simulink model "ESC_Example"  (Simulink 8.3)
settings: Solver=ode45  StartTime=0.0  StopTime=5  MaxStep=0.001  RelTol=1e-3
model workspace (MAT data in the model file):
  Cf = 38925
  Cr = 38255
  Izz = 5428
  K = 19
  X = [0 0.000200950914521 0.00120570548712 0.00622947835014 0.0313483426652 0.0646816759986 0.0980150093319 0.131348342665 0.164681675999 0.198015009332 0.231348342665 0.264681675999 ... (5155 elements, 5155x1)]
  Y = [0 0 0 0 0 0 0 0 0 0 0 0 ... (5155 elements, 5155x1)]
  deltaf = [0 0 0 0 0 0 0 0 0 0 0 0 ... (5155 elements, 5155x1)]
  frame = 100
  imanual = 0
  lf = 1.488
  lr = 1.712
  m = 2045
  mu = 0.9
  ncar = 10
  psi = [0 0 0 0 0 0 0 0 0 0 0 0 ... (5155 elements, 5155x1)]
  scale = 2
  tout = [0 6.02852743562e-06 3.61711646137e-05 0.000186884350504 0.000940450279957 0.00194045027996 0.00294045027996 0.00394045027996 0.00494045027996 0.00594045027996 0.00694045027996 0.00794045027996 ... (5155 elements, 5155x1)]
  yout = [0 0.000200950914521 0.00120570548712 0.00622947835014 0.0313483426652 0.0646816759986 0.0980150093319 0.131348342665 0.164681675999 0.198015009332 0.231348342665 0.264681675999 ... (20620 elements, 5155x4)]
PreLoadFcn:
  | load('ESC_Example.mat');
StopFcn:
  | X = yout(:,1);
  | Y = yout(:,2);
  | psi = yout(:,3);
  | deltaf = yout(:,4);
  | frame = 100;
  | imanual = 0;
  | scale = 2;
  | ncar = 10;
  | 
  | anim_tracking_ESC(X,Y,psi,tout,scale,deltaf,frame,imanual)
undefined symbols (not defined in the file): sigbuilder_block
libraries: simulink x1
settings Model: Creator=Park  LastModifiedBy=user
settings DataIOCC: LimitDataPoints=off
settings OptimizationCC: ExpressionDepthLimit=2147483647
settings DebuggingCC: FcnCallInpInsideContextMsg=UseLocalSettings  FrameProcessingCompatibilityMsg=error
settings ConfigComp: CovMetricSettings=dw  CovHtmlReporting=on  CovSaveCumulativeToWorkspaceVar=on  CovSaveSingleToWorkspaceVar=on  CovModelRefEnable=Off  CovExternalEMLEnable=off

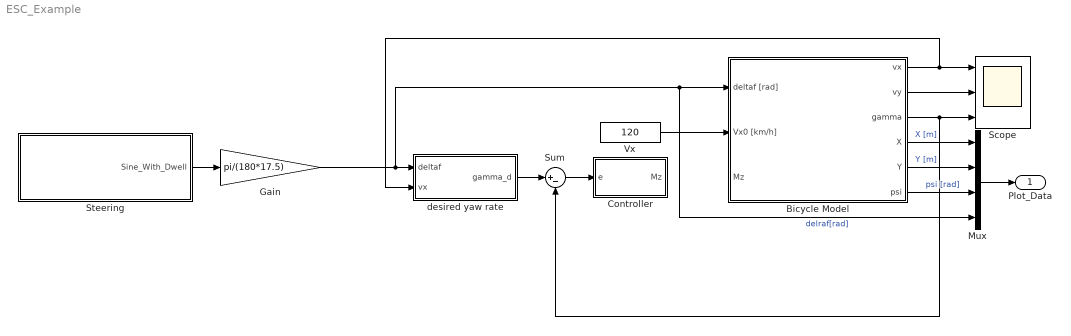
== system ESC_Example ==
  Bicycle Model : Subsystem
  Controller : Subsystem  TreatAsAtomicUnit=on
  Gain : Gain  Gain=pi/(180*17.5)
  Mux : Mux
  Scope : Scope  NumInputPorts=3
  Steering : Subsystem  Tag=STV Subsys  LoadFcn=sigbuilder_block('load');  StartFcn=sigbuilder_block('start');  StopFcn=sigbuilder_block('stop');  ClipboardFcn=sigbuilder_block('clipboard');  mask(Sigbuilder block){}
      mask help: Simulink:masks:SigbuilderBlock_MD
      mask init:
      | if ~strcmp(get_param(bdroot(gcbh),'SimulationStatus'),'stopped') tuvar = sigbuilder_block('maskInit'); end
      settings: CopyFcn=sigbuilder_block('copy');  DeleteFcn=sigbuilder_block('delete');  ModelCloseFcn=sigbuilder_block('modelClose');  PreSaveFcn=sigbuilder_block('preSave');  PauseFcn=sigbuilder_block('pause');  ContinueFcn=sigbuilder_block('continue');  NameChangeFcn=sigbuilder_block('namechange');  OpenFcn=sigbuilder_block('open',[0 29.7931 635.586 392.276 ]);  CloseFcn=sigbuilder_block('close');
      mask Display: plot(0, 0, 100, 100,[2, 2, 32, 32, 2], [68, 8, 8, 68, 68],[32, 2], [38, 38], [32, 19, 2],[53, 60, 44], [32, 17, 17, 2],[16, 16, 31, 31]);txt = getActiveGroup(gcbh);text(2, 100, txt,'verticalAlignment', 'top');
  Sum : Sum  Inputs=|+-
  Vx : Constant  Value=120
  desired yaw rate : Subsystem
  Plot_Data : Outport
  wires:
  Steering/1(Sine_With_Dwell) -> Gain/1
  Bicycle Model/4(X) -> Mux/1  "X [m]"
  Bicycle Model/5(Y) -> Mux/2  "Y [m]"
  Bicycle Model/6(psi) -> Mux/3  "psi [rad]"
  Mux/1 -> Plot_Data/1
  Bicycle Model/1(vx) -> desired yaw rate/2(vx), Scope/1
  Bicycle Model/2(vy) -> Scope/2
  Bicycle Model/3(gamma) -> Sum/2, Scope/3
  Gain/1 -> Mux/4, Bicycle Model/1(deltaf [rad]), desired yaw rate/1(deltaf)  "delraf[rad]"
  desired yaw rate/1(gamma_d) -> Sum/1
  Sum/1 -> Controller/1(e)
  Vx/1 -> Bicycle Model/2(Vx0 [km/h])

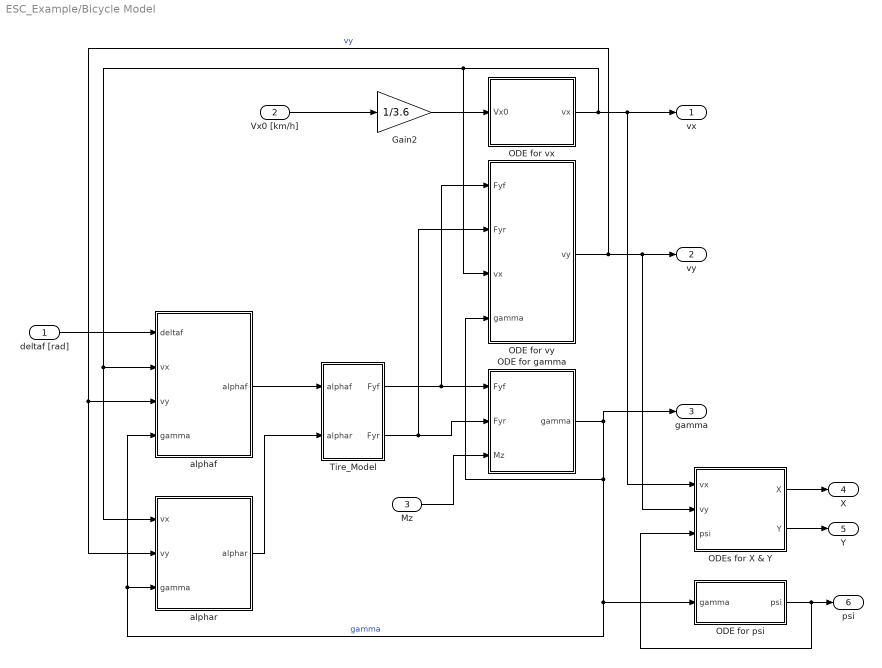
== system ESC_Example/Bicycle Model ==
  deltaf [rad] : Inport
  Vx0 [km/h] : Inport  Port=2
  Mz : Inport  Port=3
  Gain2 : Gain  Gain=1/3.6
  ODE for gamma : Subsystem
  ODE for psi : Subsystem
  ODE for vx : Subsystem
  ODE for vy : Subsystem
  ODEs for X & Y : Subsystem
  Tire_Model : Subsystem  Variant=on
  alphaf : Subsystem
  alphar : Subsystem
  vx : Outport
  vy : Outport  Port=2
  gamma : Outport  Port=3
  X : Outport  Port=4
  Y : Outport  Port=5
  psi : Outport  Port=6
  wires:
  alphaf/1(alphaf) -> Tire_Model/1(alphaf)
  alphar/1(alphar) -> Tire_Model/2(alphar)
  Tire_Model/1(Fyf) -> ODE for gamma/1(Fyf), ODE for vy/1(Fyf)
  Tire_Model/2(Fyr) -> ODE for gamma/2(Fyr), ODE for vy/2(Fyr)
  ODE for gamma/1(gamma) -> gamma/1, ODE for vy/4(gamma), alphar/3(gamma), alphaf/4(gamma), ODE for psi/1(gamma)  "gamma"
  ODE for vy/1(vy) -> ODEs for X & Y/2(vy), vy/1, alphaf/3(vy), alphar/2(vy)  "vy"
  ODE for vx/1(vx) -> alphaf/2(vx), alphar/1(vx), ODE for vy/3(vx), ODEs for X & Y/1(vx), vx/1
  ODE for psi/1(psi) -> ODEs for X & Y/3(psi), psi/1
  deltaf [rad]/1 -> alphaf/1(deltaf)
  ODEs for X & Y/1(X) -> X/1
  ODEs for X & Y/2(Y) -> Y/1
  Vx0 [km/h]/1 -> Gain2/1
  Gain2/1 -> ODE for vx/1(Vx0)
  Mz/1 -> ODE for gamma/3(Mz)

== system ESC_Example/Controller ==
  e : Inport
  PID Controller : simulink/Continuous/PID Controller  Controller=PID  TimeDomain=Continuous-time  SampleTime=-1  IntegratorMethod=Forward Euler  FilterMethod=Forward Euler  Form=Parallel  P=108153.175289364  I=433866.001986902  D=-1959.17350386418  N=55.2034697672503  InitialConditionSource=internal  InitialConditionForIntegrator=0  InitialConditionForFilter=0  ExternalReset=none  LimitOutput=off  UpperSaturationLimit=inf  LowerSaturationLimit=-inf  LinearizeAsGain=on  AntiWindupMode=none  Kb=1  TrackingMode=off  Kt=1  PParamMin=[]  PParamMax=[]  IParamMin=[]  IParamMax=[]  DParamMin=[]  DParamMax=[]  NParamMin=[]  NParamMax=[]  KbParamMin=[]  KbParamMax=[]  KtParamMin=[]  KtParamMax=[]  POutMin=[]  POutMax=[]  IOutMin=[]  IOutMax=[]  DOutMin=[]  DOutMax=[]  NOutMin=[]  NOutMax=[]  KbOutMin=[]  KbOutMax=[]  KtOutMin=[]  KtOutMax=[]  IntegratorOutMin=[]  IntegratorOutMax=[]  FilterOutMin=[]  FilterOutMax=[]  SumOutMin=[]  SumOutMax=[]  SumI1OutMin=[]  SumI1OutMax=[]  SumI2OutMin=[]  SumI2OutMax=[]  SumI3OutMin=[]  SumI3OutMax=[]  SumDOutMin=[]  SumDOutMax=[]  SaturationOutMin=[]  SaturationOutMax=[]  IntegratorContinuousStateAttributes=''  IntegratorStateMustResolveToSignalObject=off  IntegratorRTWStateStorageClass=Auto  FilterContinuousStateAttributes=''  FilterStateMustResolveToSignalObject=off  FilterRTWStateStorageClass=Auto
  Mz : Outport
  wires:
  e/1 -> PID Controller/1
  PID Controller/1 -> Mz/1

== system ESC_Example/Steering ==
  Demux : Demux  Tag=STV Demux  Outputs=1
  FromWs : FromWorkspace  Tag=STV FromWs  VariableName=tuvar  SampleTime=0  SigBuilderData=DataTag1  VnvData=DataTag2
      SigBuilderData=|
      | common.afterFinalStr = 'Extrapolate'
      | common.sampleTime = 0
      | dataSet.timeRange = [0 10]
      | dataSet.name = 'Sine_With_Dwell'
      | sbobj.Groups.Name = 'Sine_With_Dwell'
      | sbobj.Groups.Signals.Name = 'Sine_With_Dwell'
      | sbobj.Groups.Signals.XData = [0 1 1.01 1.02 1.03 1.04 1.05 1.06 1.07 1.08 1.09 1.1 1.11 1.12 1.13 1.14 1.15 1.16 1.17 1.18 1.19 1.2 1.21 1.22 1.23 1.24 1.25 1.26 1.27 1.28 1.29 1.3 1.31 1.32 1.33 1.34 1.35 1.36 1.37 1.38 1.39 1.4 1.41 1.42 1.43 1.44 1.45 1.46 1.47 1.48 1.49 1.5 1.51 1.52 1.53 1.54 1.55 1.56 1.57 1.58 1.59 1.6 1.61 1.62 1.63 1.64 1.65 1.66 1.67 1.68 1.69 1.7 1.71 1.72 1.73 1.74 1.75 1.76 1.77 1.78 1.79 1.8 1.81 1.82 1.83 1.84 1.85 1.86 1.87 1.88 1.89 1.9 1.91 1.92 1.93 1.94 1.95 1.96 1.97 1.98 1.99 2 2.01 2.02 2.03 2.04 2.05 2.06 2.07 2.071 2.57 2.58 2.59 2.6 2.61 2.62 2.63 2.64 2.65 2.66 2.67 2.68 2.69 2.7 2.71 2.72 2.73 2.74 2.75 2.76 2.77 2.78 2.79 2.8 2.81 2.82 2.83 2.84 2.85 2.86 2.87 2.88 2.89 2.9 2.91 2.92 2.927 10]
      | sbobj.Groups.Signals.YData = [0 0 11.87139195 23.71982307 35.52237696 47.25622593 58.89867518 70.4272067 81.8195228 93.05358926 104.1076779 114.9604087 125.5907911 135.9782644 146.1027381 155.9446299 165.4849046 174.7051097 183.5874123 192.1146329 200.2702787 208.0385756 215.4044987 222.3538014 228.8730428 234.9496137 240.5717616 245.7286121 250.4101914 254.6074448 258.312254 261.5174535 264.2168442 266.405205 268.0783032 269.232903 269.8667714 269.978682 269.5684185 268.6367747 267.185552 265.2175577 262.736598 259.7474714 256.2559592 252.2688144 247.7937489 242.839418 237.4154037 231.5321972 225.2011772 218.4345885 211.2455189 203.6478728 195.6563451 187.2863925 178.5542037 169.4766675 160.0713414 150.3564165 140.3506825 130.073492 119.5447224 108.7847376 97.81434902 86.65477466 75.32759864 63.85472919 52.25835638 40.56090906 28.78501166 16.95344028 5.089078724 -6.78512577 -18.64620695 -30.47122392 -42.23730557 -53.92169474 -65.50179231 -76.95520086 -88.25976801 -99.39362922 -110.3352502 -121.0634684 -131.5575339 -141.7971501 -151.762512 -161.4343455 -170.7939437 -179.8232042 -188.5046631 -196.8215294 -204.7577172 -212.2978767 -219.4274244 -226.1325708 -232.4003474 -238.2186312 -243.5761691 -248.4625988 -252.8684694 -256.7852594 -260.2053932 -263.1222557 -265.5302054 -267.4245849 -268.8017304 -269.6589783 -269.9946705 -270 -270 -269.8081577 -269.0998005 -267.8709693 -266.1240407 -263.8623933 -261.0904017 -257.8134272 -254.0378076 -249.7708458 -245.0207946 -239.7968412 -234.1090893 -227.9685399 -221.3870696 -214.3774077 -206.9531118 -199.1285417 -190.9188309 -182.3398583 -173.4082164 -164.1411804 -154.5566739 -144.6732347 -134.5099784 -124.0865624 -113.4231467 -102.5403558 -91.45923846 -80.20122702 -68.78809593 -57.24191969 -45.58503008 -33.83997306 -22.02946512 -10.17634932 0 0]
  Sine_With_Dwell : Outport  Tag=STV Outport
  wires:
  FromWs/1 -> Demux/1
  Demux/1 -> Sine_With_Dwell/1

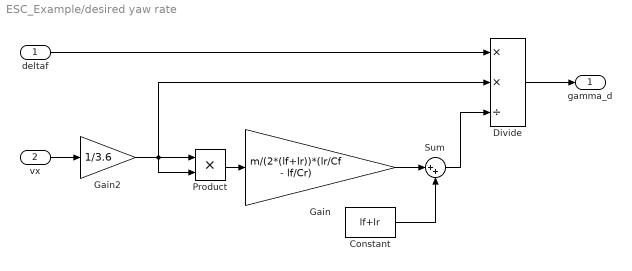
== system ESC_Example/desired yaw rate ==
  deltaf : Inport
  vx : Inport  Port=2
  Constant : Constant  Value=lf+lr
  Divide : Product  Inputs=**/
  Gain : Gain  Gain=m/(2*(lf+lr))*(lr/Cf - lf/Cr)
  Gain2 : Gain  Gain=1/3.6
  Product : Product  RndMeth=Zero
  Sum : Sum  Inputs=|++
  gamma_d : Outport
  wires:
  vx/1 -> Gain2/1
  Product/1 -> Gain/1
  Gain/1 -> Sum/1
  Constant/1 -> Sum/2
  Sum/1 -> Divide/3
  deltaf/1 -> Divide/1
  Divide/1 -> gamma_d/1
  Gain2/1 -> Product/1, Product/2, Divide/2

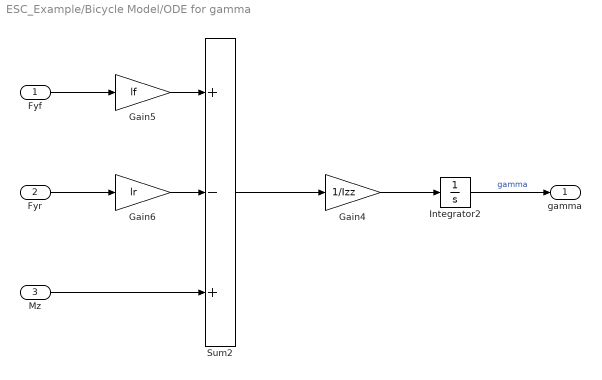
== system ESC_Example/Bicycle Model/ODE for gamma ==
  Fyf : Inport
  Fyr : Inport  Port=2
  Mz : Inport  Port=3
  Gain4 : Gain  Gain=1/Izz
  Gain5 : Gain  Gain=lf
  Gain6 : Gain  Gain=lr
  Integrator2 : Integrator  ContinuousStateAttributes='gamma'
  Sum2 : Sum  Inputs=+-+
  gamma : Outport
  wires:
  Sum2/1 -> Gain4/1
  Gain4/1 -> Integrator2/1
  Gain5/1 -> Sum2/1
  Gain6/1 -> Sum2/2
  Fyf/1 -> Gain5/1
  Integrator2/1 -> gamma/1  "gamma"
  Fyr/1 -> Gain6/1
  Mz/1 -> Sum2/3

== system ESC_Example/Bicycle Model/ODE for psi ==
  gamma : Inport
  Integrator : Integrator  ContinuousStateAttributes='psi'
  psi : Outport
  wires:
  gamma/1 -> Integrator/1  "dpsi"
  Integrator/1 -> psi/1

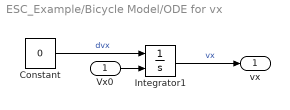
== system ESC_Example/Bicycle Model/ODE for vx ==
  Vx0 : Inport
  Constant : Constant  Value=0
  Integrator1 : Integrator  InitialConditionSource=external  InitialCondition=80/3.6  ContinuousStateAttributes='vx'
  vx : Outport
  wires:
  Constant/1 -> Integrator1/1  "dvx"
  Integrator1/1 -> vx/1  "vx"
  Vx0/1 -> Integrator1/2

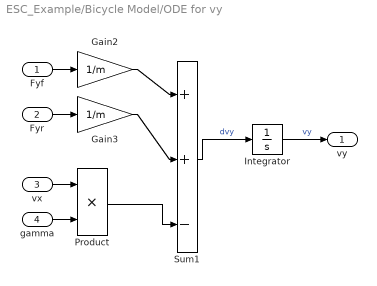
== system ESC_Example/Bicycle Model/ODE for vy ==
  Fyf : Inport
  Fyr : Inport  Port=2
  vx : Inport  Port=3
  gamma : Inport  Port=4
  Gain2 : Gain  Gain=1/m
  Gain3 : Gain  Gain=1/m
  Integrator : Integrator  ContinuousStateAttributes='vy'
  Product : Product  RndMeth=Zero
  Sum1 : Sum  Inputs=++|-
  vy : Outport
  wires:
  Gain2/1 -> Sum1/1
  Gain3/1 -> Sum1/2
  Sum1/1 -> Integrator/1  "dvy"
  Product/1 -> Sum1/3
  Fyf/1 -> Gain2/1
  Fyr/1 -> Gain3/1
  Integrator/1 -> vy/1  "vy"
  vx/1 -> Product/1
  gamma/1 -> Product/2

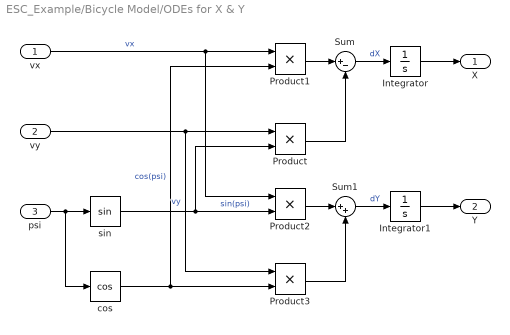
== system ESC_Example/Bicycle Model/ODEs for X & Y ==
  vx : Inport
  vy : Inport  Port=2
  psi : Inport  Port=3
  Integrator : Integrator  ContinuousStateAttributes='X'
  Integrator1 : Integrator  ContinuousStateAttributes='Y'
  Product{,1..3} (4 alike) : Product  RndMeth=Zero
  Sum : Sum  Inputs=|+-
  Sum1 : Sum  Inputs=|++
  cos : Trigonometry  Operator=cos
  sin : Trigonometry
  X : Outport
  Y : Outport  Port=2
  wires:
  psi/1 -> sin/1, cos/1
  sin/1 -> Product/2, Product2/2  "sin(psi)"
  vy/1 -> Product/1, Product3/1  "vy"
  vx/1 -> Product1/1, Product2/1  "vx"
  cos/1 -> Product1/2, Product3/2  "cos(psi)"
  Product1/1 -> Sum/1
  Product/1 -> Sum/2
  Sum/1 -> Integrator/1  "dX"
  Product2/1 -> Sum1/1
  Product3/1 -> Sum1/2
  Sum1/1 -> Integrator1/1  "dY"
  Integrator/1 -> X/1
  Integrator1/1 -> Y/1

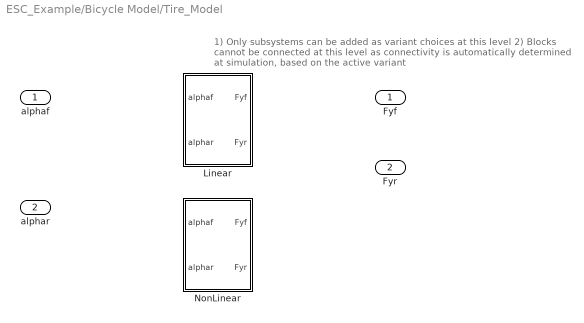
== system ESC_Example/Bicycle Model/Tire_Model ==
  note: 1) Only subsystems can be added as variant choices at this level
      | 2) Blocks cannot be connected at this level as connectivity is
      | automatically determined at simulation, based on the active variant
  alphaf : Inport
  alphar : Inport  Port=2
  Linear : Subsystem  VariantControl=Variant
  NonLinear : Subsystem  VariantControl=Variant1
  Fyf : Outport
  Fyr : Outport  Port=2

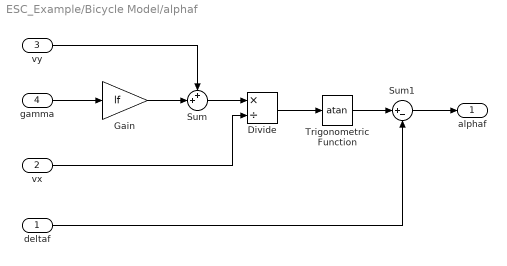
== system ESC_Example/Bicycle Model/alphaf ==
  deltaf : Inport
  vx : Inport  Port=2
  vy : Inport  Port=3
  gamma : Inport  Port=4
  Divide : Product  Inputs=*/
  Gain : Gain  Gain=lf
  Sum : Sum  Inputs=++|
  Sum1 : Sum  Inputs=|+-
  Trigonometric Function : Trigonometry  Operator=atan
  alphaf : Outport
  wires:
  gamma/1 -> Gain/1
  vy/1 -> Sum/1
  Gain/1 -> Sum/2
  Sum/1 -> Divide/1
  vx/1 -> Divide/2
  Divide/1 -> Trigonometric Function/1
  Trigonometric Function/1 -> Sum1/1
  deltaf/1 -> Sum1/2
  Sum1/1 -> alphaf/1

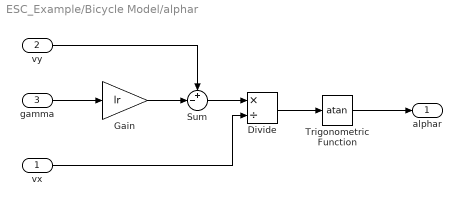
== system ESC_Example/Bicycle Model/alphar ==
  vx : Inport
  vy : Inport  Port=2
  gamma : Inport  Port=3
  Divide : Product  Inputs=*/
  Gain : Gain  Gain=lr
  Sum : Sum  Inputs=+-|
  Trigonometric Function : Trigonometry  Operator=atan
  alphar : Outport
  wires:
  Trigonometric Function/1 -> alphar/1
  Divide/1 -> Trigonometric Function/1
  vx/1 -> Divide/2
  Sum/1 -> Divide/1
  Gain/1 -> Sum/2
  vy/1 -> Sum/1
  gamma/1 -> Gain/1

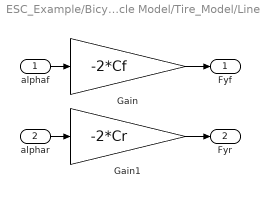
== system ESC_Example/Bicycle Model/Tire_Model/Linear ==
  alphaf : Inport
  alphar : Inport  Port=2
  Gain : Gain  Gain=-2*Cf
  Gain1 : Gain  Gain=-2*Cr
  Fyf : Outport
  Fyr : Outport  Port=2
  wires:
  alphaf/1 -> Gain/1
  Gain/1 -> Fyf/1
  alphar/1 -> Gain1/1
  Gain1/1 -> Fyr/1

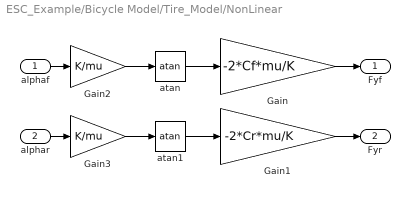
== system ESC_Example/Bicycle Model/Tire_Model/NonLinear ==
  alphaf : Inport
  alphar : Inport  Port=2
  Gain : Gain  Gain=-2*Cf*mu/K
  Gain1 : Gain  Gain=-2*Cr*mu/K
  Gain2 : Gain  Gain=K/mu
  Gain3 : Gain  Gain=K/mu
  atan : Trigonometry  Operator=atan
  atan1 : Trigonometry  Operator=atan
  Fyf : Outport
  Fyr : Outport  Port=2
  wires:
  Gain1/1 -> Fyr/1
  alphar/1 -> Gain3/1
  Gain/1 -> Fyf/1
  alphaf/1 -> Gain2/1
  Gain2/1 -> atan/1
  atan/1 -> Gain/1
  Gain3/1 -> atan1/1
  atan1/1 -> Gain1/1
